simulink library "vmc"  (R2021b)
settings: Solver=VariableStepAuto  StartTime=0.0  StopTime=10.0  RelTol=1e-3
undefined symbols (not defined in the file or in its folder): AVMC_ACCDeltaTqIGain_X_kph, AVMC_ACCDeltaTqIGain_Y_mps2, AVMC_ACCDeltaTqIGainP2_X_kph, AVMC_ACCDeltaTqIGainP2_Y_mps2, AVMC_ACCDeltaTqPGain_X_kph, AVMC_ACCDeltaTqPGain_Y_kph, AVMC_ACCDeltaTqPGainP2_X_kph, AVMC_ACCDeltaTqPGainP2_Y_kph, AVMC_ACCLongSteadyCtrl_X_kph, AVMC_CCAccelCMD_X_kph, AVMC_CCAccelCMD_Y_kph, AVMC_CCDeltaTqIGain_X_kph, AVMC_CCDeltaTqIGain_Y_mps2, AVMC_CCDeltaTqPGain_X_kph, AVMC_CCDeltaTqPGain_Y_kph, AVMC_CCLongSteadyCtrl_X_kph, AVMC_DISCDeltaTqIGainP2_X_kph, AVMC_DISCDeltaTqIGainP2_Y_mps2, AVMC_ESCRegenOut_X_kph, AVMC_ESCRegenOut_Y_Deg, AVMC_ESCRegenOutEnSpd_X_Deg, AVMC_LatESCRegenOut_X_kph, AVMC_LatESCRegenOut_Y_Deg, AVMC_LongAccDeadZone_X_kph, AVMC_LongAccDeadZoneP2_X_kph, AVMC_LongAccFiltTs_X_Gps, AVMC_LongAccFiltTsP2_X_Gps, AVMC_MCPresBaseTq_X_bar, AVMC_MSAAccelCMD_X_kph, AVMC_MSAAccelCMD_Y_kph, AVMC_MSADeltaTqIGain_X_kph, AVMC_MSADeltaTqIGain_Y_mps2, AVMC_MSADeltaTqPGain_X_kph, AVMC_MSADeltaTqPGain_Y_kph, AVMC_MSALongSteadyCtrl_X_kph, AVMC_MSAPedalOvrd_X_kph, AVMC_MSASpdBand_X_kph, AVMC_OPDDisSlideRate_X_Deg, AVMC_RDCDetectTime_X_kph, AVMC_RDCDetectTime_Y_pct, AVMC_RDCEnSlideRate_X_Deg, AVMC_StESCYaw_X_kph, AVMC_StESCYaw_Y_Deg, AVMC_StESCYawCom_X_kph, AVMC_StESCYawCom_Y_Gps, AVMC_TMSpdBaseTq_X_rpm, C_TASK_10MS_S, C_TASK_5MS_S, DEG2RAD, Discrete, ENUM_ADASACCSTA_ACTIVE, ENUM_ADASACCSTA_OVERRIDE, ENUM_ADASACCSTA_STANDBY, ENUM_ADASMSASTA_ACTIVE, ENUM_ADASMSASTA_ERROR, ENUM_ADASMSASTA_OFF, ENUM_ADASMSASTA_OVERSPEED, ENUM_ADASMSASTA_STANDBY, ENUM_ADASMSASTA_UNDERSPEED, ENUM_ADASMSASTA_UNLIMIT ... (+254)
libraries: hcu_lib x57, simulink x49, ctrlSharedLib x6, simulink_extras x1
(part 9 of 9)

== stateflow chart vmc/VMC/Subsystem1/TimeGapJudgement ==
  state TimeGapJudgement
    (default) -> (junction 11) : {VVMC_TimeGapJudge_flag = FALSE}
    TimeGapJudgement -> (junction 11)
    (junction 11) -> (junction 71) [order 1] : [(VINP_VehSpeed_kph * KPH2MPS - VINP_ACCObjRelSpd_mps) > ZERO_FLOAT]
    (junction 11) -> (junction 33) [order 2] : {VVMC_TimeGapJudge_flag = FALSE;
        |  VVMC_TimeGapCalcu_s = KVMC_TimeGapMax_s}
    (junction 71) -> (junction 24) : {VVMC_TimeGapCalcu_s = VINP_ACCObjDist_m / (VINP_VehSpeed_kph * KPH2MPS - VINP_ACCObjRelSpd_mps)}
    (junction 24) -> (junction 29) [order 1] : [VINP_TimeGapLevel_enum == ENUM_TIMEGAPLEVEL_LEVEL1]
    (junction 29) -> (junction 27) [order 1] : [VVMC_TimeGapCalcu_s <= KVMC_TimeGapBandLv1_s]
    (junction 24) -> (junction 35) [order 2]
    (junction 29) -> (junction 44) [order 2] : {VVMC_TimeGapJudge_flag = FALSE}
    (junction 27) -> (junction 31) : {VVMC_TimeGapJudge_flag = TRUE}
    (junction 35) -> (junction 38) [order 1] : [VINP_TimeGapLevel_enum == ENUM_TIMEGAPLEVEL_LEVEL2]
    (junction 38) -> (junction 42) [order 1] : [VVMC_TimeGapCalcu_s <= KVMC_TimeGapBandLv2_s]
    (junction 35) -> (junction 56) [order 2]
    (junction 38) -> (junction 46) [order 2] : {VVMC_TimeGapJudge_flag = FALSE}
    (junction 42) -> (junction 40) : {VVMC_TimeGapJudge_flag = TRUE}
    (junction 56) -> (junction 49) [order 1] : [VINP_TimeGapLevel_enum == ENUM_TIMEGAPLEVEL_LEVEL3]
    (junction 49) -> (junction 50) [order 1] : [VVMC_TimeGapCalcu_s <= KVMC_TimeGapBandLv3_s]
    (junction 56) -> (junction 59) [order 2]
    (junction 49) -> (junction 48) [order 2] : {VVMC_TimeGapJudge_flag = FALSE}
    (junction 50) -> (junction 53) : {VVMC_TimeGapJudge_flag = TRUE}
    (junction 59) -> (junction 65) [order 1] : [VINP_TimeGapLevel_enum == ENUM_TIMEGAPLEVEL_LEVEL4]
    (junction 65) -> (junction 64) [order 1] : [VVMC_TimeGapCalcu_s <= KVMC_TimeGapBandLv4_s]
    (junction 59) -> (junction 68) [order 2] : {VVMC_TimeGapJudge_flag = FALSE}
    (junction 65) -> (junction 66) [order 2] : {VVMC_TimeGapJudge_flag = FALSE}
    (junction 64) -> (junction 58) : {VVMC_TimeGapJudge_flag = TRUE}
  data: VINP_ACCObjRelSpd_mps input; VINP_ACCObjDist_m input single; VINP_VehSpeed_kph input single; KPH2MPS input single; VINP_TimeGapLevel_enum input uint8; VVMC_TimeGapJudge_flag output boolean; ENUM_TIMEGAPLEVEL_LEVEL1 input uint8; KVMC_TimeGapBandLv1_s input single; ENUM_TIMEGAPLEVEL_LEVEL2 input uint8; KVMC_TimeGapBandLv2_s input single; ENUM_TIMEGAPLEVEL_LEVEL3 input uint8; KVMC_TimeGapBandLv3_s input single; ENUM_TIMEGAPLEVEL_LEVEL4 input uint8; KVMC_TimeGapBandLv4_s input single; TRUE input boolean; FALSE input boolean; ZERO_FLOAT input single; KVMC_TimeGapMax_s input single; VVMC_TimeGapCalcu_s output single

== stateflow chart vmc/VMC/ACC_ReqAccelControl/ConstantSpeedControl1 ==
  state ConstantSpeedControl
    (default) -> (junction 2) : {SpdCtrlFlag = 0;
        |  ReqAccel = 0}
    ConstantSpeedControl -> (junction 2)
    (junction 2) -> (junction 6) [order 1] : [DeltaSpeed >= KVMC_SpdCtrlEnBand_kph && SpdCtrlFlag == 0]
    (junction 2) -> (junction 16) [order 2]
    (junction 6) -> (junction 8) : {SpdCtrlFlag = 1;
        |  ReqAccel = MINUSONE_FLOAT * KVMC_SpdCtrlReqAccel_mps2}
    (junction 16) -> (junction 15) [order 1] : [DeltaSpeed <= MINUSONE_FLOAT * KVMC_SpdCtrlEnBand_kph && SpdCtrlFlag == 0]
    (junction 16) -> (junction 20) [order 2]
    (junction 15) -> (junction 12) : {SpdCtrlFlag = 1;
        |  ReqAccel = KVMC_SpdCtrlReqAccel_mps2}
    (junction 20) -> (junction 18) [order 1] : [SpdCtrlFlag == 1]
    (junction 18) -> (junction 24) [order 1] : [ReqAccel > ZERO_FLOAT]
    (junction 24) -> (junction 26) [order 1] : [DeltaSpeed >= KVMC_SpdCtrlDisBand_kph]
    (junction 20) -> (junction 42) [order 2] : {SpdCtrlFlag = 0}
    (junction 18) -> (junction 40) [order 2]
    (junction 24) -> (junction 30) [order 2] : {SpdCtrlFlag = 1;
        |  ReqAccel = KVMC_SpdCtrlReqAccel_mps2}
    (junction 26) -> (junction 28) : {SpdCtrlFlag = 0;
        |  ReqAccel = ZERO_FLOAT}
    (junction 40) -> (junction 37) [order 1] : [ReqAccel < ZERO_FLOAT]
    (junction 37) -> (junction 33) [order 1] : [DeltaSpeed <= MINUSONE_FLOAT * KVMC_SpdCtrlDisBand_kph]
    (junction 40) -> (junction 49) [order 2]
    (junction 37) -> (junction 35) [order 2] : {SpdCtrlFlag = 1;
        |  ReqAccel = MINUSONE_FLOAT * KVMC_SpdCtrlReqAccel_mps2}
    (junction 33) -> (junction 38) : {SpdCtrlFlag = 0;
        |  ReqAccel = ZERO_FLOAT}
  data: DeltaSpeed input single; SpdCtrlFlag local boolean; ReqAccel output single; KVMC_SpdCtrlEnBand_kph input single; KVMC_SpdCtrlDisBand_kph input single; MINUSONE_FLOAT input single; KVMC_SpdCtrlReqAccel_mps2 input single; ZERO_FLOAT input single

== stateflow chart vmc/VMC/Long Acceleration Calculation/WheelSpeedRollingAverage/WheelSpeedRollingAverage ==
  state WheelSpeedRollingAverage
    (default) -> (junction 84) : {VVMC_RollAveCount_enum = ONE_INT}
    WheelSpeedRollingAverage -> (junction 84)
    (junction 84) -> (junction 7) : {VVMC_LFWhlSpeedRollAve_kph = ZERO_FLOAT;
        |  VVMC_RFWhlSpeedRollAve_kph = ZERO_FLOAT;
        |  VVMC_LRWhlSpeedRollAve_kph = ZERO_FLOAT;
        |  VVMC_RRWhlSpeedRollAve_kph = ZERO_FLOAT}
    (junction 7) -> (junction 12) [order 1] : [VVMC_RollAveCount_enum < KVMC_WhlSpdRollAveLevel_enum]
    (junction 7) -> (junction 30) [order 2]
    (junction 12) -> (junction 15) : {% Wheel Speed Memory
        |  VVMC_LFWhlSpeedMemory_kph[VVMC_RollAveCount_enum] = VINP_LFRawWhlSpeed_kph;
        |  VVMC_RFWhlSpeedMemory_kph[VVMC_RollAveCount_enum] = VINP_RFRawWhlSpeed_kph;
        |  VVMC_LRWhlSpeedMemory_kph[VVMC_RollAveCount_enum] = VINP_LRRawWhlSpeed_kph;
        |  VVMC_RRWhlSpeedMemory_kph[VVMC_RollAveCount_enum] = VINP_RRRawWhlSpeed_kph;
        |
        |  % Wheel Speed Memory Shift Counter
        |  VVMC_WhlSpeedShiftCount_enum = ONE_INT}
    (junction 15) -> (junction 66) [order 2]
    (junction 15) -> (junction 59) [order 1] : [VVMC_WhlSpeedShiftCount_enum <= VVMC_RollAveCount_enum]
    (junction 66) -> (junction 68) : {% Wheel Speed Rolling Average
        |  VVMC_LFWhlSpeedRollAve_kph = VVMC_LFWhlSpeedRollAve_kph / VVMC_RollAveCount_enum;
        |  VVMC_RFWhlSpeedRollAve_kph = VVMC_RFWhlSpeedRollAve_kph / VVMC_RollAveCount_enum;
        |  VVMC_LRWhlSpeedRollAve_kph = VVMC_LRWhlSpeedRollAve_kph / VVMC_RollAveCount_enum;
        |  VVMC_RRWhlSpeedRollAve_kph = VVMC_RRWhlSpeedRollAve_kph / VVMC_RollAveCount_enum;
        |
        |  % Rolling Average Counter
        |  VVMC_RollAveCount_enum++}
    (junction 63) -> (junction 15) : {VVMC_WhlSpeedShiftCount_enum++}
    (junction 59) -> (junction 61) : {% Wheel Speed Rolling Average
        |  VVMC_LFWhlSpeedRollAve_kph = VVMC_LFWhlSpeedRollAve_kph + VVMC_LFWhlSpeedMemory_kph[VVMC_WhlSpeedShiftCount_enum];
        |  VVMC_RFWhlSpeedRollAve_kph = VVMC_RFWhlSpeedRollAve_kph + VVMC_RFWhlSpeedMemory_kph[VVMC_WhlSpeedShiftCount_enum];
        |  VVMC_LRWhlSpeedRollAve_kph = VVMC_LRWhlSpeedRollAve_kph + VVMC_LRWhlSpeedMemory_kph[VVMC_WhlSpeedShiftCount_enum];
        |  VVMC_RRWhlSpeedRollAve_kph = VVMC_RRWhlSpeedRollAve_kph + VVMC_RRWhlSpeedMemory_kph[VVMC_WhlSpeedShiftCount_enum]}
    (junction 61) -> (junction 63)
    (junction 30) -> (junction 32) [order 1] : [VVMC_RollAveCount_enum == KVMC_WhlSpdRollAveLevel_enum]
    (junction 30) -> (junction 56) [order 2]
    (junction 32) -> (junction 79) : {% Wheel Speed Memory
        |  VVMC_LFWhlSpeedMemory_kph[VVMC_RollAveCount_enum] = VINP_LFRawWhlSpeed_kph;
        |  VVMC_RFWhlSpeedMemory_kph[VVMC_RollAveCount_enum] = VINP_RFRawWhlSpeed_kph;
        |  VVMC_LRWhlSpeedMemory_kph[VVMC_RollAveCount_enum] = VINP_LRRawWhlSpeed_kph;
        |  VVMC_RRWhlSpeedMemory_kph[VVMC_RollAveCount_enum] = VINP_RRRawWhlSpeed_kph;
        |
        |  % Wheel Speed Memory Shift Counter
        |  VVMC_WhlSpeedShiftCount_enum = ONE_INT}
    (junction 79) -> (junction 73) [order 2]
    (junction 79) -> (junction 74) [order 1] : [VVMC_WhlSpeedShiftCount_enum <= VVMC_RollAveCount_enum]
    (junction 73) -> (junction 34) : {% Wheel Speed Rolling Average
        |  VVMC_LFWhlSpeedRollAve_kph = VVMC_LFWhlSpeedRollAve_kph / VVMC_RollAveCount_enum;
        |  VVMC_RFWhlSpeedRollAve_kph = VVMC_RFWhlSpeedRollAve_kph / VVMC_RollAveCount_enum;
        |  VVMC_LRWhlSpeedRollAve_kph = VVMC_LRWhlSpeedRollAve_kph / VVMC_RollAveCount_enum;
        |  VVMC_RRWhlSpeedRollAve_kph = VVMC_RRWhlSpeedRollAve_kph / VVMC_RollAveCount_enum;
        |
        |  % Wheel Speed Memory Shift Counter
        |  VVMC_WhlSpeedShiftCount_enum = ONE_INT}
    (junction 76) -> (junction 79) : {VVMC_WhlSpeedShiftCount_enum++}
    (junction 74) -> (junction 71) : {% Wheel Speed Rolling Average
        |  VVMC_LFWhlSpeedRollAve_kph = VVMC_LFWhlSpeedRollAve_kph + VVMC_LFWhlSpeedMemory_kph[VVMC_WhlSpeedShiftCount_enum];
        |  VVMC_RFWhlSpeedRollAve_kph = VVMC_RFWhlSpeedRollAve_kph + VVMC_RFWhlSpeedMemory_kph[VVMC_WhlSpeedShiftCount_enum];
        |  VVMC_LRWhlSpeedRollAve_kph = VVMC_LRWhlSpeedRollAve_kph + VVMC_LRWhlSpeedMemory_kph[VVMC_WhlSpeedShiftCount_enum];
        |  VVMC_RRWhlSpeedRollAve_kph = VVMC_RRWhlSpeedRollAve_kph + VVMC_RRWhlSpeedMemory_kph[VVMC_WhlSpeedShiftCount_enum]}
    (junction 71) -> (junction 76)
    (junction 34) -> (junction 56) [order 2]
    (junction 34) -> (junction 37) [order 1] : [VVMC_WhlSpeedShiftCount_enum < VVMC_RollAveCount_enum]
    (junction 54) -> (junction 34) : { VVMC_WhlSpeedShiftCount_enum++}
    (junction 37) -> (junction 39) : {% Wheel Speed Memory Shift
        |  VVMC_LFWhlSpeedMemory_kph[VVMC_WhlSpeedShiftCount_enum] = VVMC_LFWhlSpeedMemory_kph[VVMC_WhlSpeedShiftCount_enum + ONE_INT];
        |  VVMC_RFWhlSpeedMemory_kph[VVMC_WhlSpeedShiftCount_enum] = VVMC_RFWhlSpeedMemory_kph[VVMC_WhlSpeedShiftCount_enum + ONE_INT];
        |  VVMC_LRWhlSpeedMemory_kph[VVMC_WhlSpeedShiftCount_enum] = VVMC_LRWhlSpeedMemory_kph[VVMC_WhlSpeedShiftCount_enum + ONE_INT];
        |  VVMC_RRWhlSpeedMemory_kph[VVMC_WhlSpeedShiftCount_enum] = VVMC_RRWhlSpeedMemory_kph[VVMC_WhlSpeedShiftCount_enum + ONE_INT];}
    (junction 39) -> (junction 54)
  data: VINP_LFRawWhlSpeed_kph input; VINP_RFRawWhlSpeed_kph input; VINP_LRRawWhlSpeed_kph input; VINP_RRRawWhlSpeed_kph input; VVMC_RollAveCount_enum local uint8 size=1; ONE_INT input; KVMC_WhlSpdRollAveLevel_enum input; VVMC_LFWhlSpeedRollAve_kph output double; VVMC_RFWhlSpeedRollAve_kph output double; VVMC_LRWhlSpeedRollAve_kph output double; VVMC_RRWhlSpeedRollAve_kph output double; VVMC_LFWhlSpeedMemory_kph local double size=300; VVMC_LRWhlSpeedMemory_kph local double size=300; VVMC_RFWhlSpeedMemory_kph local double size=300; VVMC_RRWhlSpeedMemory_kph local double size=300; VVMC_WhlSpeedShiftCount_enum local double; ZERO_FLOAT input

== stateflow chart vmc/VMC/IMU/IMU sensing result /RollingAverage1 ==
  state RollingAverage
    (default) -> (junction 2) : {VVMC_RollAveCount_enum = ONE_INT}
    RollingAverage -> (junction 2)
    (junction 2) -> (junction 3) : {VVMC_RollAve_raw32 = ZERO_FLOAT}
    (junction 3) -> (junction 100) [order 1] : [VVMC_RollAveCount_enum < KVMC_RollAveLevel_enum]
    (junction 3) -> (junction 37) [order 2]
    (junction 100) -> (junction 5) : {% Memory
        |  VVMC_Memory_raw32[VVMC_RollAveCount_enum] = VINP_INPData_raw32;
        |
        |  % Memory Shift Counter
        |  VVMC_ShiftCount_enum = ONE_INT}
    (junction 5) -> (junction 7) [order 2]
    (junction 5) -> (junction 6) [order 1] : [VVMC_ShiftCount_enum <= VVMC_RollAveCount_enum]
    (junction 7) -> (junction 8) : {% Rolling Average
        |  VVMC_RollAve_raw32 = VVMC_RollAve_raw32 / VVMC_RollAveCount_enum;
        |
        |  % Rolling Average Counter
        |  VVMC_RollAveCount_enum++}
    (junction 35) -> (junction 5) : {VVMC_ShiftCount_enum++}
    (junction 6) -> (junction 36) : {% Rolling Average Sum
        |  VVMC_RollAve_raw32 = VVMC_RollAve_raw32 + VVMC_Memory_raw32[VVMC_ShiftCount_enum];
        |  }
    (junction 36) -> (junction 35)
    (junction 37) -> (junction 76) [order 1] : [VVMC_RollAveCount_enum == KVMC_RollAveLevel_enum]
    (junction 76) -> (junction 47)
    (junction 37) -> (junction 60) [order 2]
    (junction 78) -> (junction 76)
    (junction 47) -> (junction 30) : {% Memory
        |  VVMC_Memory_raw32[VVMC_RollAveCount_enum] = VINP_INPData_raw32;
        |
        |  % Memory Shift Counter
        |  VVMC_ShiftCount_enum = ONE_INT;
        | }
    (junction 60) -> (junction 62) [order 1] : [VVMC_RollAveCount_enum > KVMC_RollAveLevel_enum]
    (junction 60) -> (junction 39) [order 2]
    (junction 62) -> (junction 66) : {VVMC_MemoryShiftCount_enum = ONE_INT}
    (junction 30) -> (junction 48) [order 2]
    (junction 30) -> (junction 22) [order 1] : [VVMC_ShiftCount_enum <= VVMC_RollAveCount_enum]
    (junction 48) -> (junction 45) : {% Rolling Average
        |  VVMC_RollAve_raw32 = VVMC_RollAve_raw32 / VVMC_RollAveCount_enum;
        |
        |  % Memory Shift Counter
        |  VVMC_ShiftCount_enum = ONE_INT}
    (junction 14) -> (junction 30) : {VVMC_ShiftCount_enum++}
    (junction 22) -> (junction 25) : {% Rolling Average Sum
        |  VVMC_RollAve_raw32 = VVMC_RollAve_raw32 + VVMC_Memory_raw32[VVMC_ShiftCount_enum]}
    (junction 66) -> (junction 82) [order 2]
    (junction 66) -> (junction 69) [order 1] : [VVMC_MemoryShiftCount_enum < VVMC_RollAveCount_enum]
    (junction 82) -> (junction 80) : {VVMC_RollAveCount_enum = KVMC_RollAveLevel_enum}
    (junction 73) -> (junction 66) : {VVMC_MemoryShiftCount_enum++}
    (junction 69) -> (junction 71) : {VVMC_Memory_raw32[VVMC_MemoryShiftCount_enum] =...
        |  VVMC_Memory_raw32[VVMC_RollAveCount_enum - KVMC_RollAveLevel_enum + VVMC_MemoryShiftCount_enum]}
    (junction 25) -> (junction 14)
    (junction 71) -> (junction 73)
    (junction 80) -> (junction 78)
    (junction 45) -> (junction 39) [order 2]
    (junction 45) -> (junction 15) [order 1] : [VVMC_ShiftCount_enum < VVMC_RollAveCount_enum]
    (junction 41) -> (junction 45) : { VVMC_ShiftCount_enum++}
    (junction 15) -> (junction 38) : {% Gy Memory Shift
        |  VVMC_Memory_raw32[VVMC_ShiftCount_enum] = VVMC_Memory_raw32[VVMC_ShiftCount_enum + ONE_INT]}
    (junction 38) -> (junction 41)
  data: KVMC_RollAveLevel_enum input uint8; VVMC_ShiftCount_enum local uint8; VVMC_RollAveCount_enum local uint8; VVMC_Memory_raw32 local single size=256; ZERO_FLOAT input single; ONE_INT input uint8; VVMC_RollAve_raw32 output single; VINP_INPData_raw32 input single; VVMC_MemoryShiftCount_enum local uint8

== stateflow chart vmc/VMC/IMU/IMU sensing result /RollingAverage2 ==
  state RollingAverage
    (default) -> (junction 2) : {VVMC_RollAveCount_enum = ONE_INT}
    RollingAverage -> (junction 2)
    (junction 2) -> (junction 3) : {VVMC_RollAve_raw32 = ZERO_FLOAT}
    (junction 3) -> (junction 100) [order 1] : [VVMC_RollAveCount_enum < KVMC_RollAveLevel_enum]
    (junction 3) -> (junction 37) [order 2]
    (junction 100) -> (junction 5) : {% Memory
        |  VVMC_Memory_raw32[VVMC_RollAveCount_enum] = VINP_INPData_raw32;
        |
        |  % Memory Shift Counter
        |  VVMC_ShiftCount_enum = ONE_INT}
    (junction 5) -> (junction 7) [order 2]
    (junction 5) -> (junction 6) [order 1] : [VVMC_ShiftCount_enum <= VVMC_RollAveCount_enum]
    (junction 7) -> (junction 8) : {% Rolling Average
        |  VVMC_RollAve_raw32 = VVMC_RollAve_raw32 / VVMC_RollAveCount_enum;
        |
        |  % Rolling Average Counter
        |  VVMC_RollAveCount_enum++}
    (junction 35) -> (junction 5) : {VVMC_ShiftCount_enum++}
    (junction 6) -> (junction 36) : {% Rolling Average Sum
        |  VVMC_RollAve_raw32 = VVMC_RollAve_raw32 + VVMC_Memory_raw32[VVMC_ShiftCount_enum];
        |  }
    (junction 36) -> (junction 35)
    (junction 37) -> (junction 76) [order 1] : [VVMC_RollAveCount_enum == KVMC_RollAveLevel_enum]
    (junction 76) -> (junction 47)
    (junction 37) -> (junction 60) [order 2]
    (junction 78) -> (junction 76)
    (junction 47) -> (junction 30) : {% Memory
        |  VVMC_Memory_raw32[VVMC_RollAveCount_enum] = VINP_INPData_raw32;
        |
        |  % Memory Shift Counter
        |  VVMC_ShiftCount_enum = ONE_INT;
        | }
    (junction 60) -> (junction 62) [order 1] : [VVMC_RollAveCount_enum > KVMC_RollAveLevel_enum]
    (junction 60) -> (junction 39) [order 2]
    (junction 62) -> (junction 66) : {VVMC_MemoryShiftCount_enum = ONE_INT}
    (junction 30) -> (junction 48) [order 2]
    (junction 30) -> (junction 22) [order 1] : [VVMC_ShiftCount_enum <= VVMC_RollAveCount_enum]
    (junction 48) -> (junction 45) : {% Rolling Average
        |  VVMC_RollAve_raw32 = VVMC_RollAve_raw32 / VVMC_RollAveCount_enum;
        |
        |  % Memory Shift Counter
        |  VVMC_ShiftCount_enum = ONE_INT}
    (junction 14) -> (junction 30) : {VVMC_ShiftCount_enum++}
    (junction 22) -> (junction 25) : {% Rolling Average Sum
        |  VVMC_RollAve_raw32 = VVMC_RollAve_raw32 + VVMC_Memory_raw32[VVMC_ShiftCount_enum]}
    (junction 66) -> (junction 82) [order 2]
    (junction 66) -> (junction 69) [order 1] : [VVMC_MemoryShiftCount_enum < VVMC_RollAveCount_enum]
    (junction 82) -> (junction 80) : {VVMC_RollAveCount_enum = KVMC_RollAveLevel_enum}
    (junction 73) -> (junction 66) : {VVMC_MemoryShiftCount_enum++}
    (junction 69) -> (junction 71) : {VVMC_Memory_raw32[VVMC_MemoryShiftCount_enum] =...
        |  VVMC_Memory_raw32[VVMC_RollAveCount_enum - KVMC_RollAveLevel_enum + VVMC_MemoryShiftCount_enum]}
    (junction 25) -> (junction 14)
    (junction 71) -> (junction 73)
    (junction 80) -> (junction 78)
    (junction 45) -> (junction 39) [order 2]
    (junction 45) -> (junction 15) [order 1] : [VVMC_ShiftCount_enum < VVMC_RollAveCount_enum]
    (junction 41) -> (junction 45) : { VVMC_ShiftCount_enum++}
    (junction 15) -> (junction 38) : {% Gy Memory Shift
        |  VVMC_Memory_raw32[VVMC_ShiftCount_enum] = VVMC_Memory_raw32[VVMC_ShiftCount_enum + ONE_INT]}
    (junction 38) -> (junction 41)
  data: KVMC_RollAveLevel_enum input uint8; VVMC_ShiftCount_enum local uint8; VVMC_RollAveCount_enum local uint8; VVMC_Memory_raw32 local single size=256; ZERO_FLOAT input single; ONE_INT input uint8; VVMC_RollAve_raw32 output single; VINP_INPData_raw32 input single; VVMC_MemoryShiftCount_enum local uint8
